simulink model "sim03"  (R2012b)
settings: Solver=ode45  StartTime=0.0  StopTime=10.0  RelTol=1e-3
settings Model: Creator=Administrator  LastModifiedBy=Administrator

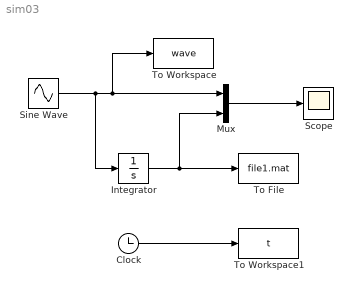
== system sim03 ==
  Clock : Clock
  Integrator : Integrator
  Mux : Mux  Inputs=2
  Scope : Scope
  Sine Wave : Sin  SampleTime=0
  To File : ToFile  Filename=file1.mat  MatrixName=wave2
  To Workspace : ToWorkspace  VariableName=wave  SampleTime=-1
  To Workspace1 : ToWorkspace  VariableName=t  SampleTime=-1
  wires:
  Sine Wave/1 -> Integrator/1, To Workspace/1, Mux/1
  Integrator/1 -> To File/1, Mux/2
  Mux/1 -> Scope/1
  Clock/1 -> To Workspace1/1
